simulink model "Multi_Scenario_WECS_based_Microgrid_2017"  (R2023a)
settings: Solver=ode45  StartTime=0.0  StopTime=4  RelTol=1e-3  EnableMultiTasking=on
undefined symbols (not defined in the file): c1, c2, c3, c4, c5, c6, DiscIntNeverNeededParam, fdesignblkfcn, gcbh, Hydride, Metal, Nickel
libraries: powerlib x63, powerlib_extras x26, powerlib_meascontrol x25, simulink x5, simulink_extras x2, electricdrivelib x1
(part 1 of 3)
settings Model: Creator=Rasool
settings SolverCC: AlgebraicLoopSolver=TrustRegion
settings DataIOCC: LimitDataPoints=on  SaveFormat=Array  ReturnWorkspaceOutputs=off
settings OptimizationCC: LifeSpan=inf
settings DebuggingCC: SolverPrmCheckMsg=warning  UnconnectedInputMsg=warning  UnconnectedOutputMsg=warning  UnconnectedLineMsg=warning  SFUnexpectedBacktrackingDiag=warning  SFNoUnconditionalDefaultTransitionDiag=warning  SFExecutionAtInitializationDiag=none  ArithmeticOperatorsInVariantConditions=warning
settings HardwareCC: ProdBitPerPointer=32  ProdBitPerSizeT=32  ProdBitPerPtrDiffT=32  ProdLargestAtomicFloat=None  ProdIntDivRoundTo=Undefined  ProdEndianess=Unspecified  ProdWordSize=32  ProdHWDeviceType=32-bit Generic
settings ModelReferenceCC: PropagateSignalLabelsOutOfModel=off
settings SFSimCC: SimUseLocalCustomCode=off  CustomCodeUndefinedFunction=UseInterfaceOnly
settings RTWCC: RTWUseLocalCustomCode=off
settings CodeAppCC: StateflowObjectComments=on
settings GRTTargetCC: TargetLangStandard=C89/C90 (ANSI)
settings ConfigComp: CovMetricSettings=dw  CovSaveCumulativeToWorkspaceVar=on  CovSaveSingleToWorkspaceVar=on  CovExternalEMLEnable=off  CovSFcnEnable=off  CovBoundaryAbsTol=1.0e-5
settings SimscapeCC: SimscapeNormalizeSystem=off

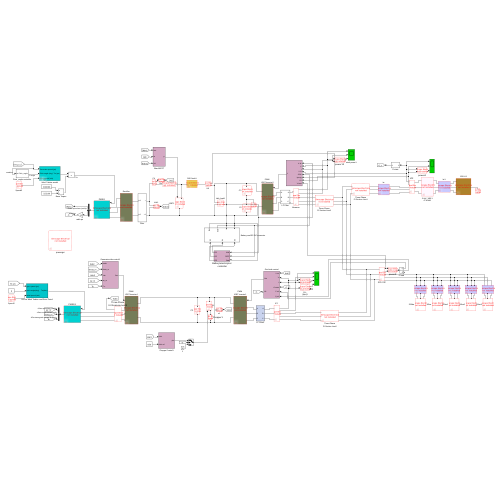
[thumbnail: Simulink's stored preview of the top-level diagram]
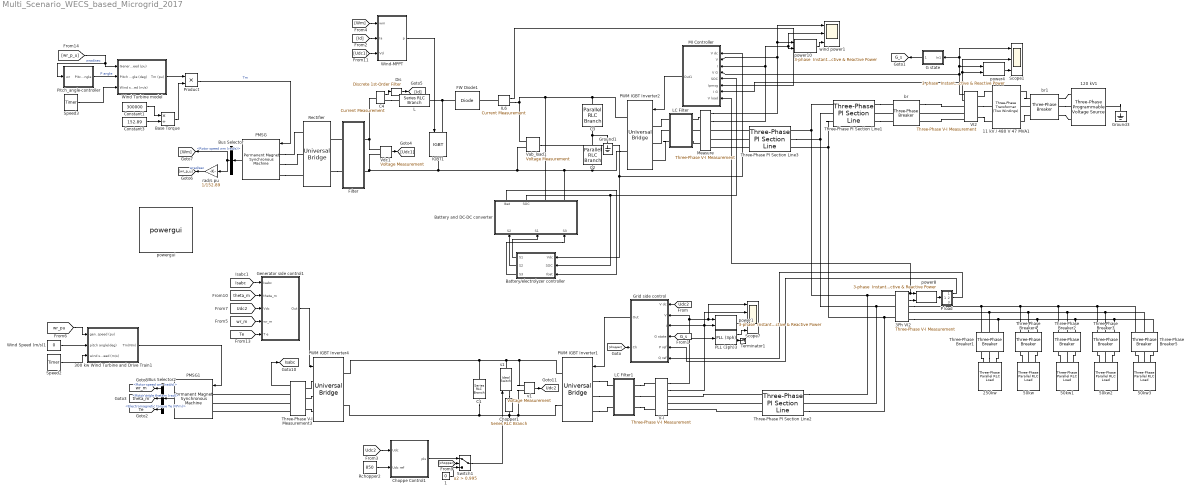
== system Multi_Scenario_WECS_based_Microgrid_2017 ==
  1 : Constant  Value=0
  11 kV / 480 V 47 MVA1 : powerlib/Elements/Three-Phase Transformer (Two Windings)  Winding1Connection=Yg  Winding2Connection=Yg  CoreType=Three single-phase transformers  SetSaturation=off  Hysteresis=off  DataFile='basic_model'  SetInitialFlux=off  Measurements=None  UNITS=SI  NominalPower=[25e6 50 ]  Winding1=[11000 0.0068652 0.00065558]  Winding2=[480 0.309217e-05 0.37449e-06]  Rm=128.72  Lm=4.0974  L0=0.5  Saturation=[0 0;17.443 34.307;3488.7 40.024]  InitialFluxes=[22.871 -22.871 20.012]  MoreParameters=off  BreakLoop=off  DataType=on  TransfoNumber=0
  120 kV1 : powerlib/Electrical Sources/Three-Phase Programmable Voltage Source  PositiveSequence=[11e3 0 50]  VariationEntity=None  VariationType=Table of time-amplitude pairs  VariationTypeAlt=Step  VariationStep=-0.2  VariationRate=10  VariationMagnitude=0.3  VariationFrequency=2  VariationTiming=[0.05 0.05+5/60]  VariationPhaseA=off  Amplitudes=[1 0.75 1.0]  TimeValues=[0 0.03 0.13]  HarmonicGeneration=off  HarmonicA=[1 -0.1 0 2]  HarmonicB=[2 0.15 35 2]*0  Timing="[0.1  2]"  BusType=swing  Pref=0  Qref=0  Qmin=-inf  Qmax=inf
  250kw : powerlib/Elements/Three-Phase Parallel RLC Load  LConnTagsString=A|B|C  Configuration=Y (grounded)  NominalVoltage=480  NominalFrequency=50  ActivePower=100e3  InductivePower=0  CapacitivePower=0  Measurements=None  LoadType=constant Z
  300 kw Wind Turbine and Drive Train1 : Subsystem
  3Ph VI2 : powerlib/Measurements/Three-Phase V-I Measurement  VoltageMeasurement=phase-to-ground  SetLabelV=off  LabelV=Vabc  Vpu=off  VpuLL=off  CurrentMeasurement=yes  SetLabelI=off  LabelI=Iabc  Ipu=off  Pbase=100e6  Vbase=480  OutputType=Complex  PhasorSimulation=off  PSBequivalent=0
  50kw{,1..3} (4 alike) : powerlib/Elements/Three-Phase Parallel RLC Load  LConnTagsString=A|B|C  Configuration=Y (grounded)  NominalVoltage=480  NominalFrequency=50  ActivePower=50e3  InductivePower=0  CapacitivePower=0  Measurements=None  LoadType=constant Z
  Base Torque : Product  Inputs=*/  RndMeth=Zero
  Battery and DC-DC converter : Subsystem
  Battery/electrolyzer controller : Subsystem
  Bus Selector : BusSelector  OutputSignals=Rotor speed wm (rad/s)
  Bus Selector2 : BusSelector  OutputSignals=Rotor speed wm (rad/s),Rotor angle thetam (rad),Electromagnetic torque Te (N*m)
  C1 : powerlib/Elements/Series RLC Branch  LConnTagsString=__new0  RConnTagsString=__new0  BranchType=C  Resistance=1  Inductance=1e-3  SetiL0=off  InitialCurrent=0  Capacitance=5000e-6  Setx0=on  InitialVoltage=800  Measurements=Branch voltage and current
  C2 : powerlib/Elements/Parallel RLC Branch  LConnTagsString=a  RConnTagsString=__new0  BranchType=C  Resistance=1.0  Inductance=1.0  SetiL0=off  InitialCurrent=0  Capacitance=5000e-6*2  Setx0=off  InitialVoltage=0  Measurements=None
  C3 : powerlib/Elements/Parallel RLC Branch  LConnTagsString=a  RConnTagsString=__new0  BranchType=C  Resistance=1.0  Inductance=1.0  SetiL0=off  InitialCurrent=0  Capacitance=5000e-6*2  Setx0=off  InitialVoltage=0  Measurements=None
  C4 : powerlib/Measurements/Current Measurement  PhasorSimulation=off  OutputType=Complex  PSBequivalent=0
  Choppe Control1 : Subsystem
  Chopper1 : powerlib/Elements/Series RLC Branch  LConnTagsString=__new0  RConnTagsString=__new0  BranchType=R  Resistance=0.027  Inductance=1e-3  SetiL0=off  InitialCurrent=0  Capacitance=1e-6  Setx0=off  InitialVoltage=0  Measurements=Branch current
  Constant1 : Constant  Value=300000
  Constant3 : Constant  Value=152.89
  Dis : powerlib_extras/Discrete  Control Blocks/Discrete 1st-Order Filter  FilterType=Lowpass  Tc=100e-3  Ts=20e-6  Initialize=off  Vac_Init=[0.8 -25 60]  Vdc_Init=-0.4  PlotResponse=off  param1=[1 500 0.1]
  FW Diode1 : powerlib/Power Electronics/Diode  Ron=0.01  Lon=0  Vf=0.8  IC=0  UseSnubber=off  Rs=100  Cs=0.1e-6  Measurements=off
  Filter : Subsystem
  G state : Subsystem
  Generator side control1 : Subsystem
  Grid side control : Subsystem
  Ground1 : powerlib/Elements/Ground  LConnTagsString=a
  Ground3 : powerlib/Elements/Ground  LConnTagsString=a
  IGBT1 : powerlib/Power Electronics/IGBT  Ron=0.001  Lon=0  Vf=1  Tf=1e-6  Tt=2e-6  IC=0  Rs=1e5  Cs=inf  Measurements=off
  IL6 : powerlib/Measurements/Current Measurement  PhasorSimulation=off  OutputType=Complex  PSBequivalent=0
  L : powerlib/Elements/Series RLC Branch  LConnTagsString=__new0  RConnTagsString=__new0  BranchType=L  Resistance=0.3  Inductance=2.2e-3  SetiL0=off  InitialCurrent=0  Capacitance=100e-6  Setx0=off  InitialVoltage=0  Measurements=None
  LC Filter : Subsystem
  LC Filter1 : Subsystem
  MI Controller : Subsystem
  Measure : powerlib/Measurements/Three-Phase V-I Measurement  VoltageMeasurement=phase-to-ground  SetLabelV=off  LabelV=V1  Vpu=off  VpuLL=off  CurrentMeasurement=yes  SetLabelI=off  LabelI=I1  Ipu=off  Pbase=5.5e3  Vbase=385  OutputType=Magnitude  PhasorSimulation=off  PSBequivalent=0
  P load : Subsystem
  PLL (3ph)3 : powerlib_meascontrol/PLL/PLL (3ph)  Fmin=30  Par_Init=[0, 50]  ParK=[180, 3200, 1]  TcD=1e-4  MaxRateChangeFreq=12  FilterCutOffFreq=25  Ts=20e-6  AGC=on
  PMSG : powerlib/Machines/Permanent Magnet Synchronous Machine  NbPhases=3  FluxDistribution=Sinusoidal  RotorType=Round  MechanicalLoad=Torque Tm  PresetModel=No  ShowDetailedParameters=on  MeasurementBus=off  Resistance=0.34  Inductance=8.5e-3  dqInductances=[0.0082 0.0082]  La=0.0009  MachineConstant=Flux linkage established by magnets (V.s)  Flux=0.46  VoltageCst=1001.2172  TorqueCst=8.28  Flat=120  Mechanical=[0.4 0.0024 12]  PolePairs=5  InitialConditions=[8,30, 10,10]  InitialConditions5ph=[0 0 0 0 0 0]  TsPowergui=0  TsBlock=-1  RefAngle=90 degrees behind phase A axis (modified Park)
  PMSG1 : powerlib/Machines/Permanent Magnet Synchronous Machine  NbPhases=3  FluxDistribution=Sinusoidal  RotorType=Round  MechanicalLoad=Torque Tm  PresetModel=No  ShowDetailedParameters=on  MeasurementBus=off  Resistance=0.25  Inductance=8.5e-3  dqInductances=[0.0082 0.0082]  La=0.00075  MachineConstant=Flux linkage established by magnets (V.s)  Flux=1  VoltageCst=2539.3191  TorqueCst=21  Flat=120  Mechanical=[2 0.0025 14 0]  PolePairs=5  InitialConditions=[17.952,0, -5.28,2.64]  InitialConditions5ph=[0 0 0 0 0 0]  TsPowergui=0  TsBlock=20e-6  RefAngle=90 degrees behind phase A axis (modified Park)
  PWM IGBT Inverter1 : powerlib/Power Electronics/Universal Bridge  Arms=3  SnubberResistance=5000e2  SnubberCapacitance=inf  Device=IGBT / Diodes  Ron=1e-3  Lon=0  ForwardVoltages="[  0.0  0.0  ]"  ForwardVoltage=.8  GTOparameters=[ 1e-6 ,1e-6 ]  IGBTparameters=[ 1e-6 , 2e-6 ]  Measurements=Device currents  Measurements_2=None  converterType=Rectifier
  PWM IGBT Inverter2 : powerlib/Power Electronics/Universal Bridge  Arms=3  SnubberResistance=5000  SnubberCapacitance=inf  Device=IGBT / Diodes  Ron=1e-3  Lon=0  ForwardVoltages="[  0.0  0.0  ]"  ForwardVoltage=.8  GTOparameters=[ 1e-6 ,1e-6 ]  IGBTparameters=[ 1e-6 , 2e-6 ]  Measurements=Device currents  Measurements_2=None  converterType=Rectifier
  PWM IGBT Inverter4 : powerlib/Power Electronics/Universal Bridge  Arms=3  SnubberResistance=5000e2  SnubberCapacitance=inf  Device=IGBT / Diodes  Ron=1e-3  Lon=0  ForwardVoltages="[  0.0  0.0  ]"  ForwardVoltage=.8  GTOparameters=[ 1e-6 ,1e-6 ]  IGBTparameters=[ 1e-6 , 2e-6 ]  Measurements=Device currents  Measurements_2=None  converterType=Rectifier
  Pitch_angle-controller : Subsystem
  Product : Product  RndMeth=Zero
  Rchopper2 : Constant  Value=850
  Rectifier : powerlib/Power Electronics/Universal Bridge  Arms=3  SnubberResistance=100  SnubberCapacitance=0.1e-6  Device=Diodes  Ron=1e-3  Lon=0  ForwardVoltages="[  0.8  0.8  ]"  ForwardVoltage=.8  GTOparameters=[ 10e-6 , 20e-6 ]  IGBTparameters=[ 1e-6 , 2e-6 ]  Measurements=Device currents  Measurements_2=None  converterType=Rectifier
  Scope1 : Scope  NumInputPorts=3
  Scope7 : Scope  NumInputPorts=4
  Speed2 : powerlib_extras/Control  Blocks/Timer  t=[0 0.5 1 1.5 2 2.5 3]  e=[9 12 10 12 9 10 12]
  Speed3 : powerlib_extras/Control  Blocks/Timer  t=[0 0.5 1.5 2.5]  e=[9 12 9 11]
  Switch1 : Switch  Criteria=u2 > Threshold  Threshold=0.995  SaturateOnIntegerOverflow=off  InputSameDT=off
  Terminator1 : Terminator
  Three-Phase PI Section Line1 : powerlib/Elements/Three-Phase PI Section Line  LConnTagsString=a|b|c  RConnTagsString=A|B|C  Frequency=50  Resistances=[ 0.007 0.01564]  Inductances="[ 0.9337e-6  1.1264e-6]"  Capacitances=[12.74e-9 7.751e-9]  Length=1
  Three-Phase PI Section Line2 : powerlib/Elements/Three-Phase PI Section Line  LConnTagsString=a|b|c  RConnTagsString=A|B|C  Frequency=50  Resistances=[ 0.007 0.01564]  Inductances="[ 0.9337e-6  1.1264e-6]"  Capacitances=[12.74e-9 7.751e-9]  Length=1
  Three-Phase PI Section Line3 : powerlib/Elements/Three-Phase PI Section Line  LConnTagsString=a|b|c  RConnTagsString=A|B|C  Frequency=50  Resistances=[ 0.007 0.01564]  Inductances="[ 0.9337e-6  1.1264e-6]"  Capacitances=[12.74e-9 7.751e-9]  Length=1
  Three-Phase V-I Measurement3 : powerlib/Measurements/Three-Phase V-I Measurement  VoltageMeasurement=no  SetLabelV=off  LabelV=Vabc  Vpu=off  VpuLL=off  CurrentMeasurement=yes  SetLabelI=off  LabelI=Iabc  Ipu=off  Pbase=100e6  Vbase=480  OutputType=Complex  PhasorSimulation=off  PSBequivalent=0
  Three-Phase Breaker1 : powerlib/Elements/Three-Phase Breaker  InitialState=closed  SwitchA=on  SwitchB=on  SwitchC=on  SwitchTimes=1000  External=off  BreakerResistance=0.001  SnubberResistance=1e6  SnubberCapacitance=inf  Measurements=None
  Three-Phase Breaker2 : powerlib/Elements/Three-Phase Breaker  InitialState=closed  SwitchA=on  SwitchB=on  SwitchC=on  SwitchTimes=2.75  External=off  BreakerResistance=0.001  SnubberResistance=1e6  SnubberCapacitance=inf  Measurements=None
  Three-Phase Breaker3 : powerlib/Elements/Three-Phase Breaker  InitialState=closed  SwitchA=on  SwitchB=on  SwitchC=on  SwitchTimes=3.25  External=off  BreakerResistance=0.001  SnubberResistance=1e6  SnubberCapacitance=inf  Measurements=None
  Three-Phase Breaker4 : powerlib/Elements/Three-Phase Breaker  InitialState=open  SwitchA=on  SwitchB=on  SwitchC=on  SwitchTimes=[1.5 2.5]  External=off  BreakerResistance=0.001  SnubberResistance=1e6  SnubberCapacitance=inf  Measurements=None
  Three-Phase Breaker5 : powerlib/Elements/Three-Phase Breaker  InitialState=closed  SwitchA=on  SwitchB=on  SwitchC=on  SwitchTimes=3.75  External=off  BreakerResistance=0.001  SnubberResistance=1e6  SnubberCapacitance=inf  Measurements=None
  "V-I " : powerlib/Measurements/Three-Phase V-I Measurement  VoltageMeasurement=phase-to-ground  SetLabelV=off  LabelV=Vabc  Vpu=off  VpuLL=off  CurrentMeasurement=yes  SetLabelI=off  LabelI=Iabc  Ipu=off  Pbase=100e6  Vbase=480  OutputType=Complex  PhasorSimulation=off  PSBequivalent=0
  VI2 : powerlib/Measurements/Three-Phase V-I Measurement  VoltageMeasurement=phase-to-ground  SetLabelV=off  LabelV=Vabc  Vpu=off  VpuLL=off  CurrentMeasurement=yes  SetLabelI=off  LabelI=Iabc  Ipu=off  Pbase=100e6  Vbase=480  OutputType=Complex  PhasorSimulation=off  PSBequivalent=0
  Vab_load1 : powerlib/Measurements/Voltage Measurement  Tag=PoWeRsYsTeMmEaSuReMeNt  PhasorSimulation=off  OutputType=Magnitude  PSBequivalent=0
  Vdc1 : powerlib/Measurements/Voltage Measurement  Tag=PoWeRsYsTeMmEaSuReMeNt  PhasorSimulation=off  OutputType=Magnitude  PSBequivalent=0
  Wind Speed (m/s)1 : Constant  Value=0
  Wind Turbine model : Subsystem  AncestorBlock=DRlib/Wind Generation/Wind Turbine  DialogController=POWERSYS.PowerSysDialog  mask(Wind Turbine){Pnom=300e3, Pelec_base=300e3/0.9, wind_base=12, P_wind_base=0.8, speed_nom=1, pitch_angle=0, DisplayTurbChar=off, c1_c6=[0.51763          116          0.4            5           21     0.006795], cp_nom=0.48, lambda_nom=8.1}
      mask prompts: Pnom "Nominal mechanical output power (W):"; Pelec_base "Base power of the electrical generator (VA):"; wind_base "Base wind speed (m/s):"; P_wind_base "Maximum power at base wind speed (pu of nominal mechanical power):"; speed_nom "Base rotational speed (p.u. of base generator speed):"; pitch_angle "Pitch angle beta to display wind-turbine power characteristics (beta >=0)  (deg):"; DisplayTurbChar "Display wind turbine power characteristics"
      mask help:
      | This block implements a variable pitch wind turbine model. The performance coefficient Cp of the turbine is the mechanical output power of the turbine divided by wind power and a function of wind speed, rotational speed, and pitch angle (beta). Cp reaches its maximum value at zero beta. Select the wind-turbine power characteristics display to plot the turbine characteristics at the specified pitch angle.
      |
      | The first input is the generator speed in per unit of the generator base speed. For a synchronous or asynchronous generator, the base speed is the synchronous speed. For a permanent-magnet generator, the base speed is defined as the speed producing nominal voltage at  no load. The second input is the blade pitch angle (beta) in degrees. The third input is the wind speed in m/s.
      |
      | The output is the torque applied to the generator shaft in per unit of the generator ratings.
      |
      | The turbine inertia must be added to the generator inertia.
      mask init:
      | %Wind turbine typical characteristic data
      | %c2=116;c3=0.4;c4=5;c5=21;
      | %Computation of c1 and c6 for lambda_nom et cpmax
      | %lambda_nom=8.1;
      | %cp_max=0.48;
      | %cp_nom=cp_max;
      | 
      | %lambda_i_nom=1/(1/lambda_nom-0.035);
      | %k_nom=-(c2*c5/lambda_i_nom-c4*c5-c2)*exp(-c5/lambda_i_nom)/lambda_nom^2;
      | %c1=cp_max/((c2/lambda_i_nom-c4)*exp(-c5/lambda_i_nom)+k_nom*lambda_nom);
      | %c6=k_nom*c1;
      | power_initmask();
      mask Help: web(psbhelp);
      mask Callback Pnom:
      | ParVisible={'on','on','on','on','on','on','on','off','off','off',};
      | set_param(gcb,'MaskVisibilities',ParVisible);
      | c1_c6=str2num(get_param(gcb,'c1_c6'));
      | c1=c1_c6(1);c2=c1_c6(2);c3=c1_c6(3);c4=c1_c6(4);c5=c1_c6(5);c6=c1_c6(6);
      mask Callback DisplayTurbChar:
      | DisplayTurbChar=get_param(gcb,'DisplayTurbChar');
      | 
      | if strcmp(DisplayTurbChar,'on')
      |     fig_num=figure;
      | 	clf(fig_num);
      | 	[speed_nom,wind_base,P_wind_base,pitch_angle]=getSPSmaskvalues(gcb,{'speed_nom','wind_base','P_wind_base','pitch_angle'});
      | 	[c1_c6,lambda_nom,cp_nom]=getSPSmaskvalues(gcb,{'c1_c6','lambda_nom','cp_nom'});
      | 	c1=c1_c6(1);c2=c1_c6(2);c3=c1_c6(3);c4=c1_c6(4);c5=c1_c6(5);c6=c1_c6(6);
      | 
      | 	%Wind turbine typical characteristic data
      |     %c2=116;c3=0.4;c4=5;c5=21;
      |     %Computation of c1 and c6 for lambda_nom et cpmax
      |     %lambda_nom=8.1;
      |     %cp_max=0.48;
      |     %cp_nom=cp_max;
      | 
      |     %lambda_i_nom=1/(1/lambda_nom-0.035);
      |     %k_nom=-(c2*c5/lambda_i_nom-c4*c5-c2)*exp(-c5/lambda_i_nom)/lambda_nom^2;
      |     %c1=cp_max/((c2/lambda_i_nom-c4)*exp(-c5/lambda_i_nom)+k_nom*lambda_nom);
      |     %c6=k_nom*c1;
      | 
      | 	wr_elec_pu=1e-3:0.01:1.5;;
      |     wr_mec_pu=wr_elec_pu/speed_nom;
      |     wind_max=ceil((1.2/P_wind_base)^(1/3)*wind_base);
      |     wind_min=round(((0.1)/P_wind_base)^(1/3)*wind_base);
      |     wind1=wind_min:(wind_base-wind_min)/5:wind_base;
      |     wind2=wind_base+(wind_base-wind_min)/5:(wind_base-wind_min)/5:wind_max;
      |     wind_pu=[wind1 wind2]/wind_base;
      | 
      |     for k=1:length(wind_pu)
      |         for i=1:length(wr_mec_pu);
      |             lambda_pu=wr_mec_pu(i)/wind_pu(k);
      |             lambda=lambda_pu*lambda_nom;
      |             lambda_i=1/(1/(lambda+0.08*pitch_angle)-0.035/(pitch_angle^3+1));
      |             cp=c1*(c2/lambda_i-c3*pitch_angle-c4)*exp(-c5/lambda_i)+c6*lambda;
      |             cp_pu=cp/cp_nom;
      |             Pwind_pu(k,i)=wind_pu(k)^3*cp_pu*P_wind_base;
      |         end
      |     end
      |     for k=1:length(wind_pu)
      |         plot(wr_elec_pu,Pwind_pu(k,:))
      |         hold on
      |     end
      | 
      |     plot([speed_nom,speed_nom,0],[0,P_wind_base,P_wind_base],'r--')
      |     text(speed_nom+0.01,0+0.05,sprintf('%0.4g pu',speed_nom))
      |     text(0.01,P_wind_base+0.05,sprintf('Max. power at base wind speed (%0.4g m/s) and beta = 0 deg',wind_base))
      |     for i=1:length(wind_pu),
      |         p_max(i)=max(Pwind_pu(i,:));
      |         speed(i)=wr_elec_pu(find(Pwind_pu(i,:)==p_max(i)));
      |         text(speed(i),p_max(i),sprintf('%0.4g m/s',wind_pu(i)*wind_base))
      |     end
      |     plot([0 max(wr_elec_pu)],[0 0],'--')
      | 
      |     xlabel('Turbine speed (pu of nominal generator speed)')
      |     ylabel('Turbine output power (pu of nominal mechanical power)')
      |     title(sprintf('Turbine Power Characteristics (Pitch angle beta = %0.4g deg)',pitch_angle))
      |     axis([0 max(wr_elec_pu) min(Pwind_pu(1,:)) max(P_wind_base+0.1,max(wind_pu)^3*P_wind_base+0.1)])
      |     set_param(gcb,'DisplayTurbChar','off')
      | end
      mask Display: disp('');
  Wind-MPPT : Subsystem
  br : powerlib/Elements/Three-Phase Breaker  InitialState=closed  SwitchA=on  SwitchB=on  SwitchC=on  SwitchTimes=2  External=off  BreakerResistance=0.00001  SnubberResistance=1e6  SnubberCapacitance=inf  Measurements=None
  br1 : powerlib/Elements/Three-Phase Breaker  InitialState=closed  SwitchA=on  SwitchB=on  SwitchC=on  SwitchTimes=2  External=off  BreakerResistance=0.00001  SnubberResistance=1e6  SnubberCapacitance=inf  Measurements=None
  power{1,4,8,10} (4 alike) : powerlib_extras/Measurements/3-phase  Instantaneous  Active & Reactive Power
  powergui : powerlib/powergui  SimulationMode=Discrete  SolverType=Tustin/Backward Euler (TBE)  SampleTime=20e-6  frequency=60  SPID=off  DisableSnubberDevices=off  DisableRonSwitches=off  DisableVfSwitches=off  SwTol=0  DisplayEquations=off  Interpol=off  methode=off  Ts=0  FunctionMessages=off  echomessages=off  HookPort=off  EnableUseOfTLC=off  x0status=blocks  frequencyindice=0  Pbase=100e6  ErrMax=1e-4  Iterations=50  UnitsV=kV  UnitsW=MW  buscounter=0  RestoreLinks=warning  ResistiveCurrentMeasurement=off  Frange=[0:2:500]  Ylog=off  Xlog=on  ShowGrid=off  save=off  variable=ZData  structure=ScopeData8  ZoomFFT=off  StartTime=3  cycles=10  DisplayStyle=2  fundamental=5  FreqAxis=on  MaxFrequency=1000  frequencyindicesteady=1  RmsSteady=1  display=off
  rad/s pu : Gain  Gain=1/152.89  SaturateOnIntegerOverflow=on  OutDataTypeStr=Inherit: Same as input  ParamDataTypeStr=Inherit: Same as input
  s1 : powerlib/Power Electronics/Ideal Switch  Ron=0.001  Lon=0  IC=0  Rs=1e5  Cs=inf  Measurements=off
  v1 : powerlib/Measurements/Voltage Measurement  PhasorSimulation=off  OutputType=Complex  PSBequivalent=0
  wind power1 : Scope  NumInputPorts=3
  tag scope: G_s=global, Isabc=global, Te=global, Udc2=global, theta_m=global, wr_m=global
  wires:
  "V-I "/2 -> Grid side control/3(I), Scope7/2, power1/2
  "V-I "/1 -> PLL (3ph)3/1, Scope7/1, power1/1, Grid side control/2(V)
  Grid side control/1(Out) -> PWM IGBT Inverter1/1
  PLL (3ph)3/1 -> Scope7/4
  PLL (3ph)3/2 -> Terminator1/1
  power1/1 -> Scope7/3
  [Udc2] -> Grid side control/1(V dc)
  [G_s] -> Grid side control/4(G state)
  Grid side control/2(Ch) -> [chopper]
  G state/1(Out1) -> [G_s]
  v1/1 -> [Udc2]
  Generator side control1/1(Out) -> PWM IGBT Inverter4/1
  [Isabc] -> Generator side control1/1(Isabc)
  [theta_m] -> Generator side control1/2(theta_m)
  [Udc2] -> Generator side control1/3(Vdc)
  [wr_m] -> Generator side control1/4(wr_m)
  PMSG1/1 -> Bus Selector2/1
  Bus Selector2/1 -> [wr_m]  "<Rotor speed wm (rad/s)>"
  Bus Selector2/2 -> [theta_m]  "<Rotor angle thetam (rad)>"
  Bus Selector2/3 -> [Te]  "<Electromagnetic torque Te (N*m)>"
  [Te] -> Generator side control1/5(T e)
  [wr_pu] -> 300 kw Wind Turbine and Drive Train1/1(gen. speed (pu))
  300 kw Wind Turbine and Drive Train1/1(Tm(Nm)) -> PMSG1/1
  Wind Speed (m/s)1/1 -> 300 kw Wind Turbine and Drive Train1/2(pitch angle(deg))
  [Udc2] -> Choppe Control1/1(Udc)
  Rchopper2/1 -> Choppe Control1/2(Udc ref)
  Switch1/1 -> s1/1
  Three-Phase V-I Measurement3/1 -> [Isabc]
  [chopper] -> Switch1/2
  1/1 -> Switch1/3
  Speed2/1 -> 300 kw Wind Turbine and Drive Train1/3(wind speed (m/s))
  Choppe Control1/1(pls) -> Switch1/1
  Vab_load1/1 -> MI Controller/1(V dc), Battery/electrolyzer controller/1(Vdc)
  Battery and DC-DC converter/2(SOC) -> Battery/electrolyzer controller/2(SOC), MI Controller/5(SOC)
  Battery and DC-DC converter/1(Ibat) -> Battery/electrolyzer controller/3(Ibat)
  Battery/electrolyzer controller/2(S2) -> Battery and DC-DC converter/1(S2)
  Battery/electrolyzer controller/1(S1) -> Battery and DC-DC converter/2(S1)
  MI Controller/1(Out1) -> PWM IGBT Inverter2/1
  [Udc1] -> Wind-MPPT/3(Vd)
  [Id] -> Wind-MPPT/2(Ia)
  [Wm] -> Wind-MPPT/1(wm)
  Wind-MPPT/1(p) -> IGBT1/1
  Battery/electrolyzer controller/3(S3) -> Battery and DC-DC converter/3("S3 ")
  Measure/2 -> power10/2, wind power1/2, MI Controller/3(I)
  power10/1 -> wind power1/3
  IL6/1 -> MI Controller/6(Ipmsg)
  Measure/1 -> wind power1/1, power10/1, MI Controller/2(V)
  power4/1 -> Scope1/3
  VI2/1 -> MI Controller/4(V G), power4/1, G state/1(In1), Scope1/1
  VI2/2 -> MI Controller/7(I G), Scope1/2, power4/2
  Wind Turbine model/1(Tm (pu)) -> Product/1
  Constant1/1 -> Base Torque/1
  Constant3/1 -> Base Torque/2
  Bus Selector/1 -> [Wm], rad/s pu/1  "<Rotor speed wm (rad/s)>"
  [wr_p_u] -> Pitch_angle-controller/1(wr), Wind Turbine model/1(Generator speed (pu))  "wrad/sec"
  Product/1 -> PMSG/1  "Tm"
  Base Torque/1 -> Product/2
  Vdc1/1 -> [Udc1]
  Pitch_angle-controller/1(Pitch_angle) -> Wind Turbine model/2(Pitch angle (deg))  "P angle"
  Speed3/1 -> Wind Turbine model/3(Wind speed (m/s))
  PMSG/1 -> Bus Selector/1
  C4/1 -> Dis/1
  Dis/1 -> [Id]
  rad/s pu/1 -> [wr_p_u]  "wrad/sec"
  3Ph VI2/2 -> power8/2
  3Ph VI2/1 -> MI Controller/8(V load), power8/1
  power8/1 -> P load/1(L)
  P load/1(P) -> Grid side control/5(P ref)
  P load/2(Q) -> Grid side control/6(Q ref)
  connections:
  Three-Phase PI Section Line2/RConn1 -- "V-I "/RConn1
  Three-Phase PI Section Line2/RConn3 -- "V-I "/RConn3
  Three-Phase PI Section Line2/RConn2 -- "V-I "/RConn2
  PWM IGBT Inverter1/LConn2 -- LC Filter1/LConn2
  PWM IGBT Inverter1/LConn3 -- LC Filter1/LConn3
  LC Filter1/RConn1 -- "V-I "/LConn1
  LC Filter1/RConn3 -- "V-I "/LConn3
  LC Filter1/RConn2 -- "V-I "/LConn2
  PWM IGBT Inverter1/LConn1 -- LC Filter1/LConn1
  Three-Phase PI Section Line3/RConn3 -- 3Ph VI2/LConn3 -- Three-Phase PI Section Line2/LConn3 -- Three-Phase PI Section Line1/RConn3
  PWM IGBT Inverter1/RConn2 -- v1/LConn2 -- Chopper1/RConn1 -- PWM IGBT Inverter4/RConn2 -- C1/RConn1
  v1/LConn1 -- PWM IGBT Inverter1/RConn1 -- s1/RConn1 -- PWM IGBT Inverter4/RConn1 -- C1/LConn1
  Three-Phase V-I Measurement3/LConn1 -- PWM IGBT Inverter4/LConn1
  s1/LConn1 -- Chopper1/LConn1
  Three-Phase V-I Measurement3/LConn3 -- PWM IGBT Inverter4/LConn3
  Three-Phase V-I Measurement3/RConn3 -- PMSG1/LConn3
  Three-Phase V-I Measurement3/RConn1 -- PMSG1/LConn1
  Three-Phase V-I Measurement3/LConn2 -- PWM IGBT Inverter4/LConn2
  Three-Phase V-I Measurement3/RConn2 -- PMSG1/LConn2
  Three-Phase PI Section Line2/LConn1 -- 3Ph VI2/LConn1 -- Three-Phase PI Section Line1/RConn1 -- Three-Phase PI Section Line3/RConn1
  Vab_load1/LConn1 -- IL6/RConn1 -- Battery and DC-DC converter/RConn1 -- PWM IGBT Inverter2/RConn1 -- C3/LConn1
  Ground1/LConn1 -- C2/LConn1 -- C3/RConn1
  L/LConn1 -- IGBT1/LConn1 -- FW Diode1/LConn1
  PWM IGBT Inverter2/RConn2 -- C2/RConn1 -- Battery and DC-DC converter/RConn2 -- Vab_load1/LConn2 -- Vdc1/LConn2 -- Filter/RConn2 -- IGBT1/RConn1
  Filter/RConn1 -- C4/LConn1 -- Vdc1/LConn1
  LC Filter/RConn1 -- Measure/LConn1
  Measure/LConn2 -- LC Filter/RConn2
  Measure/LConn3 -- LC Filter/RConn3
  50kw/LConn3 -- Three-Phase Breaker4/LConn3
  LC Filter/LConn1 -- PWM IGBT Inverter2/LConn1
  50kw/LConn1 -- Three-Phase Breaker4/LConn1
  IL6/LConn1 -- FW Diode1/RConn1
  C4/RConn1 -- L/RConn1
  LC Filter/LConn3 -- PWM IGBT Inverter2/LConn3
  LC Filter/LConn2 -- PWM IGBT Inverter2/LConn2
  50kw/LConn2 -- Three-Phase Breaker4/LConn2
  Three-Phase PI Section Line3/LConn1 -- Measure/RConn1
  Three-Phase PI Section Line3/LConn2 -- Measure/RConn2
  Three-Phase PI Section Line3/LConn3 -- Measure/RConn3
  Three-Phase Breaker1/LConn2 -- 250kw/LConn2
  Three-Phase Breaker1/LConn3 -- 250kw/LConn3
  Three-Phase Breaker1/LConn1 -- 250kw/LConn1
  VI2/LConn3 -- 11 kV / 480 V 47 MVA1/RConn3
  Three-Phase PI Section Line1/LConn3 -- br/RConn3
  br1/RConn1 -- 11 kV / 480 V 47 MVA1/LConn1
  VI2/RConn3 -- br/LConn3
  Ground3/LConn1 -- 120 kV1/LConn1
  br1/RConn3 -- 11 kV / 480 V 47 MVA1/LConn3
  br/LConn1 -- VI2/RConn1
  br1/RConn2 -- 11 kV / 480 V 47 MVA1/LConn2
  Three-Phase PI Section Line1/LConn1 -- br/RConn1
  br1/LConn2 -- 120 kV1/RConn2
  11 kV / 480 V 47 MVA1/RConn1 -- VI2/LConn1
  br1/LConn3 -- 120 kV1/RConn3
  br/RConn2 -- Three-Phase PI Section Line1/LConn2
  br1/LConn1 -- 120 kV1/RConn1
  VI2/LConn2 -- 11 kV / 480 V 47 MVA1/RConn2
  VI2/RConn2 -- br/LConn2
  PMSG/LConn2 -- Rectifier/LConn2
  PMSG/LConn1 -- Rectifier/LConn1
  PMSG/LConn3 -- Rectifier/LConn3
  Filter/LConn1 -- Rectifier/RConn1
  Rectifier/RConn2 -- Filter/LConn2
  Three-Phase PI Section Line1/RConn2 -- Three-Phase PI Section Line3/RConn2 -- 3Ph VI2/LConn2 -- Three-Phase PI Section Line2/LConn2
  3Ph VI2/RConn1 -- Three-Phase Breaker1/RConn1 -- Three-Phase Breaker3/RConn1 -- Three-Phase Breaker5/RConn1 -- Three-Phase Breaker2/RConn1 -- Three-Phase Breaker4/RConn1
  Three-Phase Breaker1/RConn2 -- Three-Phase Breaker5/RConn2 -- Three-Phase Breaker3/RConn2 -- Three-Phase Breaker2/RConn2 -- Three-Phase Breaker4/RConn2 -- 3Ph VI2/RConn2
  3Ph VI2/RConn3 -- Three-Phase Breaker5/RConn3 -- Three-Phase Breaker3/RConn3 -- Three-Phase Breaker2/RConn3 -- Three-Phase Breaker4/RConn3 -- Three-Phase Breaker1/RConn3
  50kw1/LConn2 -- Three-Phase Breaker2/LConn2
  50kw1/LConn1 -- Three-Phase Breaker2/LConn1
  50kw1/LConn3 -- Three-Phase Breaker2/LConn3
  50kw2/LConn2 -- Three-Phase Breaker3/LConn2
  50kw2/LConn3 -- Three-Phase Breaker3/LConn3
  50kw2/LConn1 -- Three-Phase Breaker3/LConn1
  50kw3/LConn2 -- Three-Phase Breaker5/LConn2
  50kw3/LConn3 -- Three-Phase Breaker5/LConn3
  50kw3/LConn1 -- Three-Phase Breaker5/LConn1

== system Multi_Scenario_WECS_based_Microgrid_2017/300 kw Wind Turbine and Drive Train1 ==
  note: Turbine and Drive Train
  gen. speed (pu) : Inport
  pitch angle(deg) : Inport  Port=2
  wind speed (m/s) : Inport  Port=3
  Drive Train : Subsystem  mask(Wind Turbine shaft){H_WT=0.42, Ksh=4, D_mutual=1.4, shaft_base_speed=2*pi*60/14, w_wt0=1, torque0=0.9, Ts=20e-6}
      mask prompts: H_WT "Wind turbine inertia constant H (s):"; Ksh "Shaft spring constant (pu of nominal mechanical torque/rad):"; D_mutual "Shaft mutual damping (pu of nominal mechanical torque/pu dw):"; shaft_base_speed "Shaft base speed (rad/s):"; w_wt0 "Turbine initial speed (pu of base speed):"; torque0 "Initial output torque (pu of nominal mechanical torque):"; Ts "Sample time (s):"
      mask help:
      | This block implements a wind turbine drive train model. All shaft parameters are referred to high-speed shaft (generator shaft).
      |
      | The first input is the wind turbine torque in per unit (pu) based on the nominal power of the turbine and the base speed of the generator. The second input is the generator speed in pu based on the base speed of the generator.
      |
      | The outputs are:
      | 1- the transmitted torque of the shaft in pu based on the nominal power of the turbine and the base speed of the generator.
      | 2- the wind turbine speed in pu of the base speed of the generator.
  Power base for the Generator : Gain  Gain=-300e3/0.9/(2*pi*60/14)  SaturateOnIntegerOverflow=on  SampleTime=20e-6  OutDataTypeStr=Inherit: Same as input  ParamDataTypeStr=Inherit: Same as input
  Wind Turbine : Subsystem  mask(Wind Turbine){Pmec=300e3/0.9, wind_base=12, wind0=12, Ts=20e-6}
      mask prompts: Pmec "Nominal mechanical output power (W):"; wind_base "Base wind speed (m/s):"; wind0 "Initial wind speed (m/s):"; Ts "Sample time (s):"
      mask help:
      | This block implements a generic wind turbine models.
      |
      | The first input is the turbine speed in per unit of the generator base speed. For a synchronous or asynchronous generator, the base speed is the synchronous speed. For a permanent-magnet generator, the base speed is defined as the speed producing nominal voltage at  no load. The second input is the blade pitch angle in degrees. The third input is the wind speed in m/s.
      |
      | The output is the torque applied to the drive train in per unit based on the nominal power of the turbine and the base speed of the generator.
      mask init:
      | c1 = 0.6450;
      | c2 = 116;
      | c3 = .4;
      | c4 = 5;
      | c5 = 21;
      | c6 = .00912;  % Set Pmin in stall condition (does not vary with wind_speed_Pmax)
      | c7 = .08;
      | c8 = .035;
      | theta=0;
      | CpMax=.5;
      | lambda_CpMax=9.9495;
      | 
      | c1_c8=[c1 c2 c3 c4 c5 c6 c7 c8];
      |   
      | 
      | %   Cp = c1*(c6*lambda + (-c4 - c3*(2.5 + theta) + c2*(1/(lambda + ...
      | %   c7*(2.5 + theta)) - c8/(1 + (2.5 + theta)^3)))/exp(c5*(1/(lambda + ...
      | %   c7*(2.5 + theta)) - c8/(1 + (2.5 + theta)^3))))
      | 
      | 
      |         %%%%%%%%%%%%%%%%%%%%%%%%%%%%%%%%%%%%%%%%%%%%%%%%%%%%%%%%%%%%%%%%%%%%%%%%%%%
      |         % Operation at Cp max
      |         %%%%%%%%%%%%%%%%%%%%%%%%%%%%%%%%%%%%%%%%%%%%%%%%%%%%%%%%%%%%%%%%%%%%%%%%%%%
      |         
      |         rated_omegar=1;
      |         omegar = rated_omegar;
      |         
      |         % Enforce boundaries on wind speed
      |         % A warning could be displayed
      |         if wind_base < 6
      |             wind_base=6;
      |             disp('Warning: Wind speed at nominal speed and at Cp max has been set to 6 m/s')
      |         end
      |         if wind_base > 30
      |             wind_base=30;
      |             disp('Warning: Wind speed at nominal speed and at Cp max has been set to 30 m/s')
      |         end
      | 
      |         K1=lambda_CpMax/omegar*wind_base;
      |         
      |         % Calculation of K2 needed to get P equal to the requested value at
      |         % Cp max for the requested wind speed
      |         
      |         Prated=Pmec;
      |         P_rated_omegar_theta_zero=0.9;
      |         
      |         K2 = P_rated_omegar_theta_zero*Prated/(wind_base^3*CpMax);
      |         
      |         K1_K2=[K1 K2];
      |         
      |         %%%%%%%%%%%%%%%%%%%%%%%%%%%%%%%%%%%%%%%%%%%%%%%%%%%%%%%%%%%%%%%%%%%%%%%%%%%
      |         % End of calculation for operation at Cp max
      |         %%%%%%%%%%%%%%%%%%%%%%%%%%%%%%%%%%%%%%%%%%%%%%%%%%%%%%%%%%%%%%%%%%%%%%%%%%%
      |         
      | 
      | %%%%%%%%%%%%%%%%%%%%%%%%%%%%%%%%%%%%%%%%%%%%%%%%%%%%%%%%%%%%%%%%%%%%%%%%%%%
      | % Plot turbine characteristics
      | %%%%%%%%%%%%%%%%%%%%%%%%%%%%%%%%%%%%%%%%%%%%%%%%%%%%%%%%%%%%%%%%%%%%%%%%%%%
      settings: OpenFcn=power_openblockproxy();
      mask Display: disp('');
  Tm(Nm) : Outport
  wires:
  Wind Turbine/1(Tt (pu)) -> Drive Train/1(T_wt (pu))
  Drive Train/2(T_shaft (pu)) -> Power base for the Generator/1
  Drive Train/1(W_wt (pu)) -> Wind Turbine/1(W_wt (pu))
  pitch angle(deg)/1 -> Wind Turbine/2(Pitch angle (deg))
  wind speed (m/s)/1 -> Wind Turbine/3(Wind speed (m/s))
  Power base for the Generator/1 -> Tm(Nm)/1
  gen. speed (pu)/1 -> Drive Train/2(Generator speed (pu))

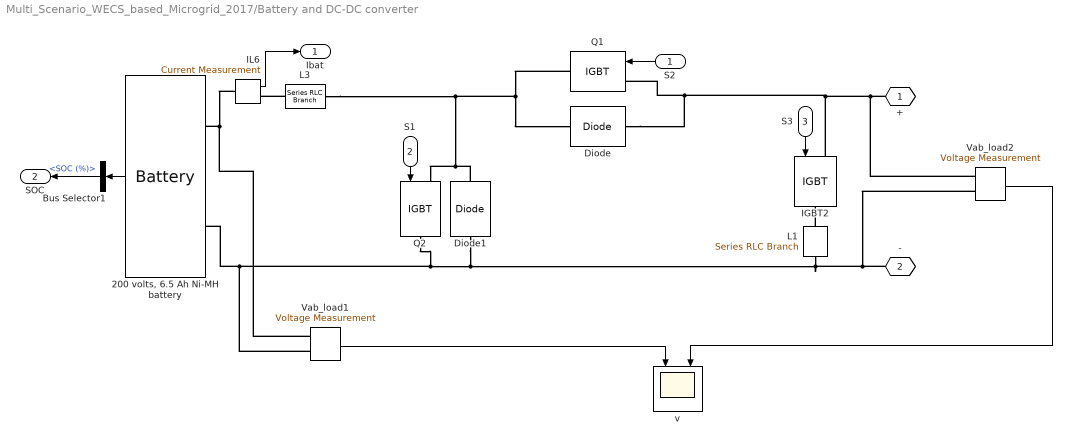
== system Multi_Scenario_WECS_based_Microgrid_2017/Battery and DC-DC converter ==
  S2 : Inport
  S1 : Inport  Port=2
  "S3 " : Inport  Port=3
  "200 volts, 6.5 Ah Ni-MH battery " : electricdrivelib/Extra Sources/Battery  BatType=Nickel-Metal-Hydride  ShowDetailedParameters=off  NomV=600  NomQ=400  SOC=60  PresetModel=on  MaxQ=430.7692  FullV=706.7797  Dis_rate=80  R=0.015  Normal_OP=384.6154  expZone="[650.8475            80]"  current=[6.5 13 32.5]  Units=Time  Batt_Tr=30
  Bus Selector1 : BusSelector  OutputSignals=SOC (%)
  Diode : powerlib/Power Electronics/Diode  Ron=0.001  Lon=0  Vf=0.8  IC=0  UseSnubber=off  Rs=500  Cs=250e-9  Measurements=off
  Diode1 : powerlib/Power Electronics/Diode  Ron=0.001  Lon=0  Vf=0.8  IC=0  UseSnubber=off  Rs=500  Cs=250e-9  Measurements=off
  IGBT2 : powerlib/Power Electronics/IGBT  Ron=0.001  Lon=0  Vf=1  Tf=1e-6  Tt=2e-6  IC=0  Rs=1e5  Cs=inf  Measurements=off
  IL6 : powerlib/Measurements/Current Measurement  PhasorSimulation=off  OutputType=Complex  PSBequivalent=0
  L1 : powerlib/Elements/Series RLC Branch  LConnTagsString=__new0  RConnTagsString=__new0  BranchType=R  Resistance=19  Inductance=2e-3  SetiL0=off  InitialCurrent=0  Capacitance=1.0  Setx0=off  InitialVoltage=0  Measurements=None
  L3 : powerlib/Elements/Series RLC Branch  LConnTagsString=__new0  RConnTagsString=__new0  BranchType=L  Resistance=1.0  Inductance=5e-3  SetiL0=off  InitialCurrent=0  Capacitance=1.0  Setx0=off  InitialVoltage=0  Measurements=None
  Q1 : powerlib/Power Electronics/IGBT  Ron=0.001  Lon=0  Vf=1  Tf=1e-6  Tt=2e-6  IC=0  Rs=1e5  Cs=inf  Measurements=off
  Q2 : powerlib/Power Electronics/IGBT  Ron=0.001  Lon=0  Vf=1  Tf=1e-6  Tt=2e-6  IC=0  Rs=1e5  Cs=inf  Measurements=off
  Vab_load1 : powerlib/Measurements/Voltage Measurement  Tag=PoWeRsYsTeMmEaSuReMeNt  PhasorSimulation=off  OutputType=Magnitude  PSBequivalent=0
  Vab_load2 : powerlib/Measurements/Voltage Measurement  Tag=PoWeRsYsTeMmEaSuReMeNt  PhasorSimulation=off  OutputType=Magnitude  PSBequivalent=0
  v : Scope  NumInputPorts=2
  + : PMIOPort  Tag=PMCPort  Side=Right
  - : PMIOPort  Tag=PMCPort  Port=2  Side=Right
  Ibat : Outport
  SOC : Outport  Port=2
  wires:
  "200 volts, 6.5 Ah Ni-MH battery "/1 -> Bus Selector1/1
  Bus Selector1/1 -> SOC/1  "<SOC (%)>"
  S2/1 -> Q1/1
  S1/1 -> Q2/1
  IL6/1 -> Ibat/1
  "S3 "/1 -> IGBT2/1
  Vab_load1/1 -> v/1
  Vab_load2/1 -> v/2
  connections:
  IL6/LConn1 -- Vab_load1/LConn1 -- "200 volts, 6.5 Ah Ni-MH battery "/LConn1
  Vab_load2/LConn2 -- -/RConn1 -- L1/RConn1 -- Diode1/LConn1 -- Q2/RConn1 -- Vab_load1/LConn2 -- "200 volts, 6.5 Ah Ni-MH battery "/LConn2
  +/RConn1 -- Vab_load2/LConn1 -- Diode/RConn1 -- Q1/LConn1 -- IGBT2/LConn1
  Diode1/RConn1 -- Diode/LConn1 -- Q1/RConn1 -- L3/RConn1 -- Q2/LConn1
  L3/LConn1 -- IL6/RConn1
  L1/LConn1 -- IGBT2/RConn1

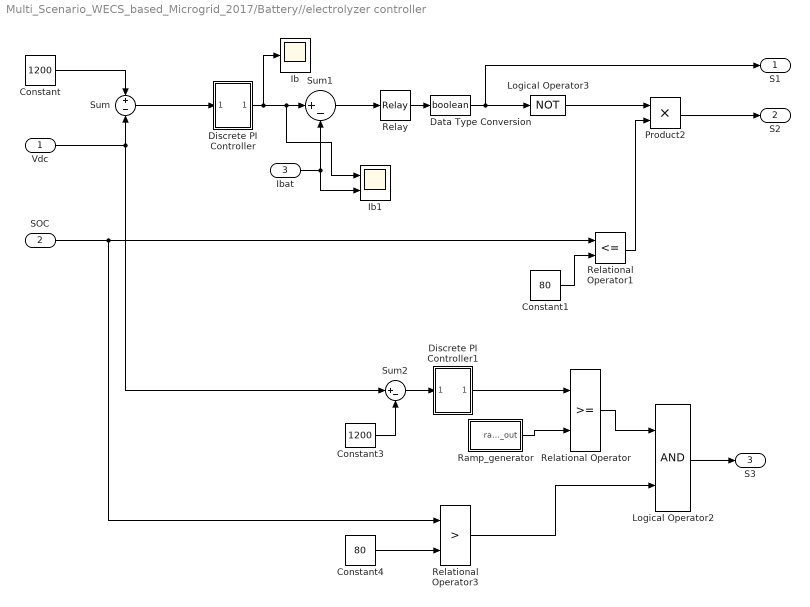
== system Multi_Scenario_WECS_based_Microgrid_2017/Battery//electrolyzer controller ==
  Vdc : Inport
  SOC : Inport  Port=2
  Ibat : Inport  Port=3
  Constant : Constant  Value=1200
  Constant1 : Constant  Value=80
  Constant3 : Constant  Value=1200
  Constant4 : Constant  Value=80
  Data Type Conversion : DataTypeConversion  OutDataTypeStr=boolean  RndMeth=Simplest
  Discrete PI Controller : Subsystem  AncestorBlock=|  DialogController=POWERSYS.PowerSysDialog  mask(Discrete PI Controller){Kp=2, Ki=60, Par_Limits=[400  -400], Init=0, Ts=20e-6}
      | powerlib_extras/Discrete 
      | Control Blocks/Discrete
      | PI Controller
      mask prompts: Kp "Proportional gain (Kp):"; Ki "Integral gain (Ki):"; Par_Limits "Output limits: [ Upper   Lower ]"; Init "Output initial value:"; Ts "Sample time:"
      mask help: This block implements a discrete PI controller.
      mask init:
      | UpperLimit=Par_Limits(1);
      | LowerLimit=Par_Limits(2);
      | power_initmask();
      mask Help: This block is part of a subset of blocks in the Extras library that does not have documentation associated with it, other than the block mask description.
      mask Display: disp('PI');
  Discrete PI Controller1 : Subsystem  AncestorBlock=|  DialogController=POWERSYS.PowerSysDialog  mask(Discrete PI Controller){Kp=60, Ki=550, Par_Limits=[1  -1], Init=0, Ts=20e-6}
      | powerlib_extras/Discrete 
      | Control Blocks/Discrete
      | PI Controller
      mask prompts: Kp "Proportional gain (Kp):"; Ki "Integral gain (Ki):"; Par_Limits "Output limits: [ Upper   Lower ]"; Init "Output initial value:"; Ts "Sample time:"
      mask help: This block implements a discrete PI controller.
      mask init:
      | UpperLimit=Par_Limits(1);
      | LowerLimit=Par_Limits(2);
      | power_initmask();
      mask Help: This block is part of a subset of blocks in the Extras library that does not have documentation associated with it, other than the block mask description.
      mask Display: disp('PI');
  Ib : Scope
  Ib1 : Scope  NumInputPorts=2
  Logical Operator2 : Logic
  Logical Operator3 : Logic  Operator=NOT
  Product2 : Product  RndMeth=Zero
  Ramp_generator : Subsystem
  Relational Operator : RelationalOperator
  Relational Operator1 : RelationalOperator  Operator=<=
  Relational Operator3 : RelationalOperator  Operator=>
  Relay : Relay  OnSwitchValue=2  OffSwitchValue=-2  OutDataTypeStr=Inherit: Inherit via back propagation
  Sum : Sum  Inputs=+-  InputSameDT=on  SaturateOnIntegerOverflow=on  OutDataTypeStr=Inherit: Same as first input
  Sum1 : Sum  Inputs=|+-  InputSameDT=on
  Sum2 : Sum  Inputs=|+-  InputSameDT=on  SaturateOnIntegerOverflow=on  OutDataTypeStr=Inherit: Same as first input
  S1 : Outport
  S2 : Outport  Port=2
  S3 : Outport  Port=3
  wires:
  Sum/1 -> Discrete PI Controller/1(Error)
  Constant/1 -> Sum/1
  Relay/1 -> Data Type Conversion/1
  Ibat/1 -> Sum1/2, Ib1/2
  Sum1/1 -> Relay/1
  Data Type Conversion/1 -> S1/1, Logical Operator3/1
  Relational Operator1/1 -> Product2/2
  Constant1/1 -> Relational Operator1/2
  Logical Operator3/1 -> Product2/1
  Product2/1 -> S2/1
  Relational Operator/1 -> Logical Operator2/1
  Constant3/1 -> Sum2/2
  Sum2/1 -> Discrete PI Controller1/1(Error)
  Ramp_generator/1(ramp_out) -> Relational Operator/2
  Discrete PI Controller1/1(Out) -> Relational Operator/1
  Vdc/1 -> Sum2/1, Sum/2
  Relational Operator3/1 -> Logical Operator2/2
  SOC/1 -> Relational Operator3/1, Relational Operator1/1
  Constant4/1 -> Relational Operator3/2
  Logical Operator2/1 -> S3/1
  Discrete PI Controller/1(Out) -> Ib/1, Ib1/1, Sum1/1

== system Multi_Scenario_WECS_based_Microgrid_2017/Choppe Control1 ==
  Udc : Inport
  Udc ref : Inport  Port=2
  "0-1 " : Saturate  UpperLimit=1  LowerLimit=0  ZeroCross=off  SampleTime=20e-6
  Discrete PI Controller : powerlib_extras/Discrete  Control Blocks/Discrete PI Controller  Kp=0.01  Ki=2  Par_Limits=[inf -inf]  Init=0  Ts=20e-6
  Divide1 : Product  Inputs=**/
  Math Function : Math  Operator=square  SignedPower=on  SampleTime=20e-6
  Math Function1 : Math  Operator=square  SignedPower=on  SampleTime=20e-6
  Pulse Generator : Subsystem  mask{Freq_sawtooth=2500, Ts=20e-6}
      mask prompts: Freq_sawtooth "Frequency of the carrier (sawtooth signal) (Hz):"; Ts "Sample time (Ts) (s):"
  Rchopper : Constant  Value=0.027
  Scope1 : Scope  NumInputPorts=2
  Scope5 : Scope  NumInputPorts=2
  Sum : Sum  Inputs=|+-
  Unit Delay1 : UnitDelay  SampleTime=20e-6  HasFrameUpgradeWarning=on
  pls : Outport
  wires:
  Sum/1 -> Discrete PI Controller/1
  Math Function/1 -> Sum/1, Scope5/1, Divide1/3
  Math Function1/1 -> Scope5/2, Sum/2
  Discrete PI Controller/1 -> Scope1/1, Divide1/2
  Rchopper/1 -> Divide1/1
  Udc/1 -> Math Function/1
  Divide1/1 -> "0-1 "/1
  Udc ref/1 -> Math Function1/1
  "0-1 "/1 -> Unit Delay1/1
  Unit Delay1/1 -> Scope1/2, Pulse Generator/1(Duty_Cycle)
  Pulse Generator/1(Pulse) -> pls/1

== system Multi_Scenario_WECS_based_Microgrid_2017/Filter ==
  C1 : powerlib/Elements/Parallel RLC Branch  LConnTagsString=a  RConnTagsString=__new0  BranchType=C  Resistance=1.0  Inductance=1.0  SetiL0=off  InitialCurrent=0  Capacitance=2000e-6  Setx0=off  InitialVoltage=650  Measurements=None
  L2 : powerlib/Elements/Series RLC Branch  LConnTagsString=__new0  RConnTagsString=__new0  BranchType=L  Resistance=1.0  Inductance=2e-3  SetiL0=off  InitialCurrent=0  Capacitance=1.0  Setx0=off  InitialVoltage=0  Measurements=None
  in1 : PMIOPort  Side=Left
  in2 : PMIOPort  Port=2  Side=Left
  + : PMIOPort  Tag=PMCPort  Port=3  Side=Right
  +1 : PMIOPort  Tag=PMCPort  Port=4  Side=Right
  connections:
  in2/RConn1 -- +1/RConn1 -- C1/RConn1
  C1/LConn1 -- +/RConn1 -- L2/RConn1
  L2/LConn1 -- in1/RConn1

== system Multi_Scenario_WECS_based_Microgrid_2017/G state ==
  In1 : Inport
  Logical Operator : Logic  Operator=NOT  AllPortsSameDT=off  OutDataTypeStr=boolean
  PLL (3ph)3 : powerlib_meascontrol/PLL/PLL (3ph)  Fmin=45  Par_Init=[0, 50]  ParK=[180, 3200, 1]  TcD=1e-4  MaxRateChangeFreq=12  FilterCutOffFreq=25  Ts=2e-05  AGC=on
  Selector Vd Vq3 : Selector  InputPortWidth=3  IndexOptions=Index vector (dialog)  Indices=[1 2]  OutputSizes=1
  Switch2 : Subsystem
  Terminator2 : Terminator
  abc to dq3 : powerlib_meascontrol/Transformations/abc to dq0  Alignment=90 degrees behind phase A axis
  Out1 : Outport
  wires:
  abc to dq3/1 -> Selector Vd Vq3/1
  In1/1 -> abc to dq3/1, PLL (3ph)3/1
  Selector Vd Vq3/1 -> Switch2/1(Vdq)
  PLL (3ph)3/2 -> abc to dq3/2
  PLL (3ph)3/1 -> Terminator2/1
  Switch2/1(SW) -> Logical Operator/1
  Logical Operator/1 -> Out1/1
